simulink model "booster_stability"  (R2024b)
settings: Solver=VariableStepAuto  StartTime=0.0  StopTime=10.0  RelTol=1e-3
values from neighbouring files (symbols this model uses):
  a = pi*r^2    (= 78.5398163397)    [script_project.m]
  Cd = 1.2    [script_project.m]
  du0 = [0, 0, 0]'    [script_project.m]
  dz0 = [0, 0, theta_tip+10, 0]'    [script_project.m]
  g = 9.81    [script_project.m]
  h = 70    [script_project.m]
  J = (1/12)*m*(b^2 + h^2)    (= 208333333.333)    [script_project.m]
  m = 500000    [script_project.m]
  rho = 1.225    [script_project.m]
  u0 = [u1eq u2eq u3eq]'    [script_project.m]
  z0 = [x2eq x2doteq thetaeq thetadoteq]'    [script_project.m]
settings Model: Creator=martinhaugen  LastModifiedBy=martinhaugen

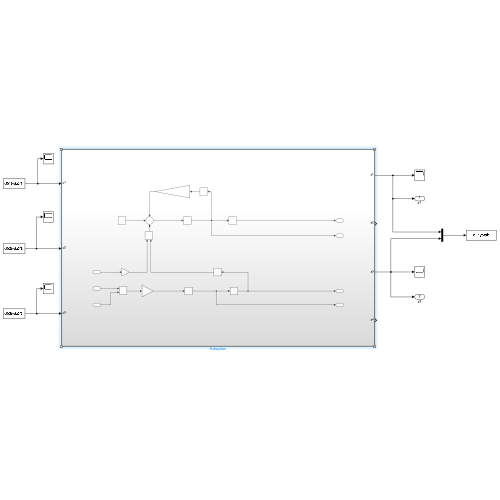
[thumbnail: Simulink's stored preview of the top-level diagram]
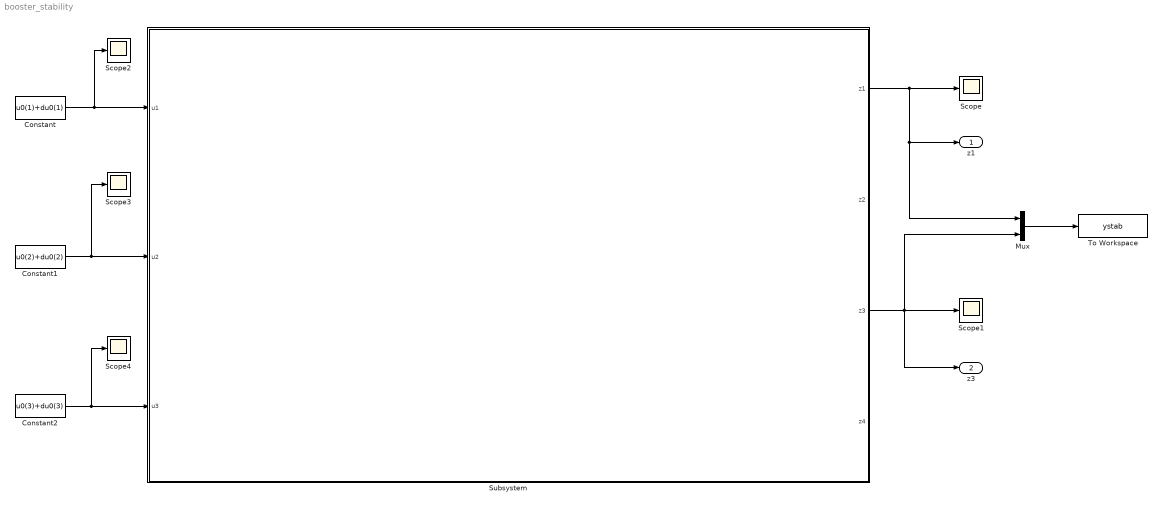
== system booster_stability ==
  Constant : Constant  Value=u0(1)+du0(1)  SampleTime=-1
  Constant1 : Constant  Value=u0(2)+du0(2)  SampleTime=-1
  Constant2 : Constant  Value=u0(3)+du0(3)  SampleTime=-1
  Mux : Mux  Inputs=2
  Scope{,1..4} (5 alike) : Scope
  Subsystem : Subsystem
  To Workspace : ToWorkspace  VariableName=ystab  SaveFormat=Timeseries  SampleTime=-1
  z1 : Outport
  z3 : Outport  Port=2
  wires:
  Constant1/1 -> Scope3/1, Subsystem/2(u2)
  Subsystem/1(z1) -> Mux/1, z1/1, Scope/1
  Subsystem/3(z3) -> Mux/2, Scope1/1, z3/1
  Constant/1 -> Scope2/1, Subsystem/1(u1)
  Constant2/1 -> Scope4/1, Subsystem/3(u3)
  Mux/1 -> To Workspace/1

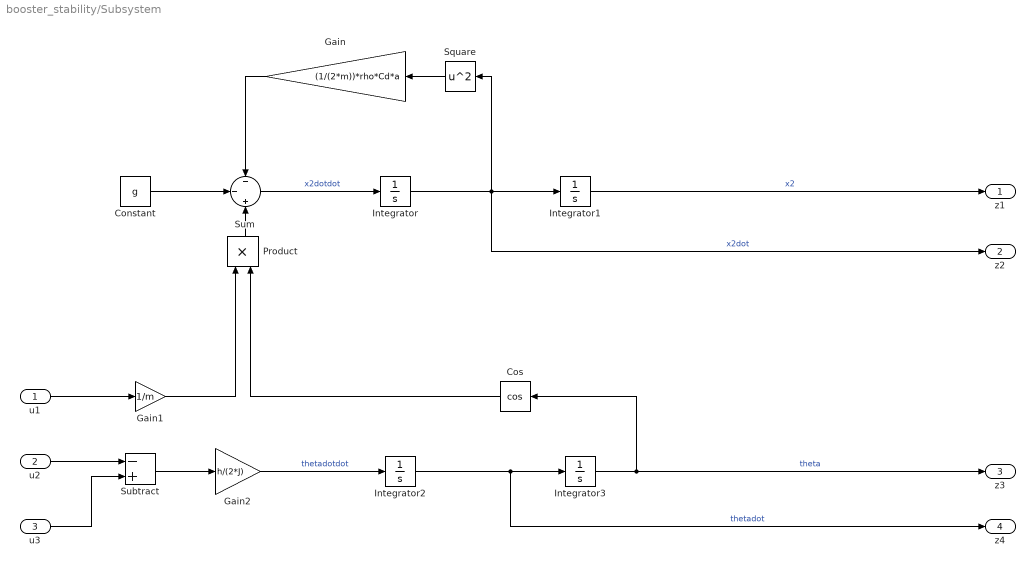
== system booster_stability/Subsystem ==
  u1 : Inport
  u2 : Inport  Port=2
  u3 : Inport  Port=3
  Constant : Constant  Value=g
  Cos : Trigonometry  Operator=cos
  Gain : Gain  Gain=(1/(2*m))*rho*Cd*a
  Gain1 : Gain  Gain=1/m
  Gain2 : Gain  Gain=h/(2*J)
  Integrator : Integrator  InitialCondition=z0(2)+dz0(2)  ContinuousStateAttributes='z2'
  Integrator1 : Integrator  InitialCondition=z0(1)+dz0(1)  ContinuousStateAttributes='z1'
  Integrator2 : Integrator  InitialCondition=z0(4)+dz0(4)  ContinuousStateAttributes='z4'
  Integrator3 : Integrator  InitialCondition=z0(3)+dz0(3)  ContinuousStateAttributes='z3'
  Product : Product
  Square : Math  Operator=square
  Subtract : Sum  Inputs=-+
  Sum : Sum  Inputs=-|-|+
  z1 : Outport
  z2 : Outport  Port=2
  z3 : Outport  Port=3
  z4 : Outport  Port=4
  wires:
  u2/1 -> Subtract/1
  Constant/1 -> Sum/2
  Square/1 -> Gain/1
  Product/1 -> Sum/3
  Subtract/1 -> Gain2/1
  Integrator/1 -> z2/1, Integrator1/1, Square/1  "x2dot"
  Gain2/1 -> Integrator2/1  "thetadotdot"
  Cos/1 -> Product/2
  u3/1 -> Subtract/2
  Integrator2/1 -> z4/1, Integrator3/1  "thetadot"
  u1/1 -> Gain1/1
  Gain/1 -> Sum/1
  Sum/1 -> Integrator/1  "x2dotdot"
  Gain1/1 -> Product/1
  Integrator3/1 -> z3/1, Cos/1  "theta"
  Integrator1/1 -> z1/1  "x2"
